simulink model "GateTestHarness_C"  (R2016a)
settings: Solver=FixedStepDiscrete  StartTime=0.0  StopTime=120  FixedStep=0.001  RelTol=1e-3
undefined symbols (not defined in the file or in its folder): sigbuilder_block
libraries: simulink x8
settings Model: Creator=omaro  LastModifiedBy=oelkawok
settings OptimizationCC: DefaultParameterBehavior=Inlined  OptimizeModelRefInitCode=on  LifeSpan=1
settings HardwareCC: ProdLongLongMode=on
settings RTWCC: SystemTargetFile=ert.tlc  TemplateMakefile=ert_default_tmf  GenerateReport=on  IncludeHyperlinkInReport=on  LaunchReport=on  GenerateTraceInfo=on  GenerateTraceReport=on  GenerateTraceReportSl=on  GenerateTraceReportSf=on  GenerateTraceReportEml=on
settings CodeAppCC: ForceParamTrailComments=on  IgnoreCustomStorageClasses=off  OperatorAnnotations=on  SimulinkDataObjDesc=on  SFDataObjDesc=on  MATLABFcnDesc=on  InsertBlockDesc=on  MATLABSourceComments=on
settings ERTTargetCC: GenerateSampleERTMain=on  InlinedParameterPlacement=NonHierarchical  ERTCustomFileTemplate=example_file_process.tlc

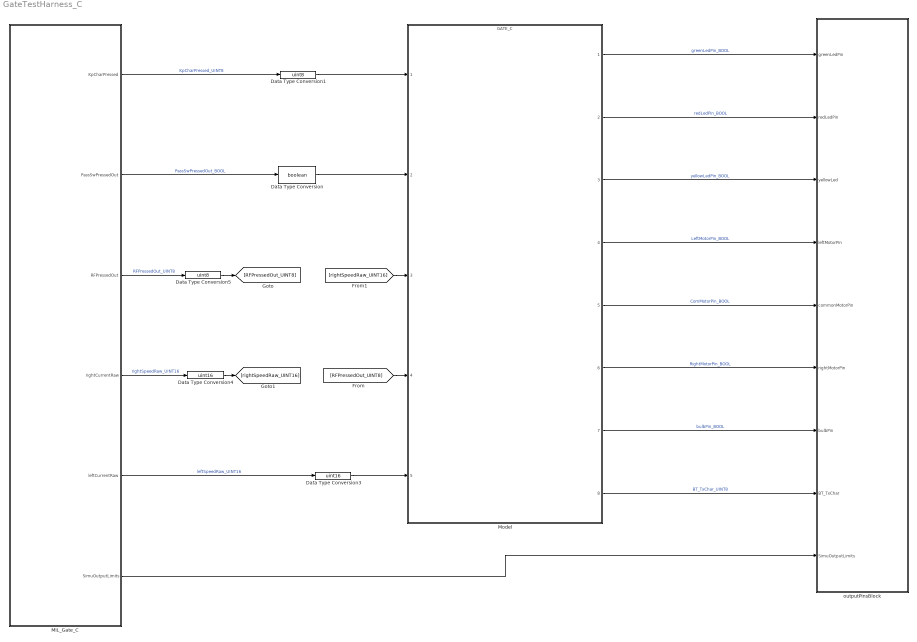
== system GateTestHarness_C ==
  Data Type Conversion : DataTypeConversion  OutDataTypeStr=boolean
  Data Type Conversion1 : DataTypeConversion  OutDataTypeStr=uint8
  Data Type Conversion3 : DataTypeConversion  OutDataTypeStr=uint16
  Data Type Conversion4 : DataTypeConversion  OutDataTypeStr=uint16
  Data Type Conversion5 : DataTypeConversion  OutDataTypeStr=uint8
  MIL_Gate_C : Subsystem  VariantControl=MIL_VariantC
  Model : ModelReference  ModelNameDialog=GATE_C.slx  SimulationMode=Normal  ModelReferenceVersion=1.328
  outputPinsBlock : Subsystem  Variant=on  VariantControl=Variant1  OverrideUsingVariant=VVOutputs
  wires:
  MIL_Gate_C/6(SimuOutputLimits) -> outputPinsBlock/9(SimuOutputLimits)
  Model/1 -> outputPinsBlock/1(greenLedPin)  "greenLedPin_BOOL"
  Model/2 -> outputPinsBlock/2(redLedPin)  "redLedPin_BOOL"
  Model/3 -> outputPinsBlock/3(yellowLed)  "yellowLedPin_BOOL"
  Model/4 -> outputPinsBlock/4(leftMotorPin)  "LeftMotorPin_BOOL"
  Model/5 -> outputPinsBlock/5(commonMotorPin)  "ComMotorPin_BOOL"
  Model/6 -> outputPinsBlock/6(rightMotorPin)  "RightMotorPin_BOOL"
  Model/7 -> outputPinsBlock/7(bulbPin)  "bulbPin_BOOL"
  Model/8 -> outputPinsBlock/8(BT_TxChar)  "BT_TxChar_UINT8"
  MIL_Gate_C/2(PassSwPressedOut) -> Data Type Conversion/1  "PassSwPressedOut_BOOL"
  MIL_Gate_C/4(rightCurrentRaw) -> Data Type Conversion4/1  "rightSpeedRaw_UINT16"
  MIL_Gate_C/3(RFPressedOut) -> Data Type Conversion5/1  "RFPressedOut_UINT8"
  MIL_Gate_C/5(leftCurrentRaw) -> Data Type Conversion3/1  "leftSpeedRaw_UINT16"
  MIL_Gate_C/1(KpCharPressed) -> Data Type Conversion1/1  "KpCharPressed_UINT8"
  Data Type Conversion1/1 -> Model/1
  Data Type Conversion3/1 -> Model/5
  Data Type Conversion/1 -> Model/2
  Data Type Conversion5/1 -> [RFPressedOut_UINT8]
  [RFPressedOut_UINT8] -> Model/4
  Data Type Conversion4/1 -> [rightSpeedRaw_UINT16]
  [rightSpeedRaw_UINT16] -> Model/3

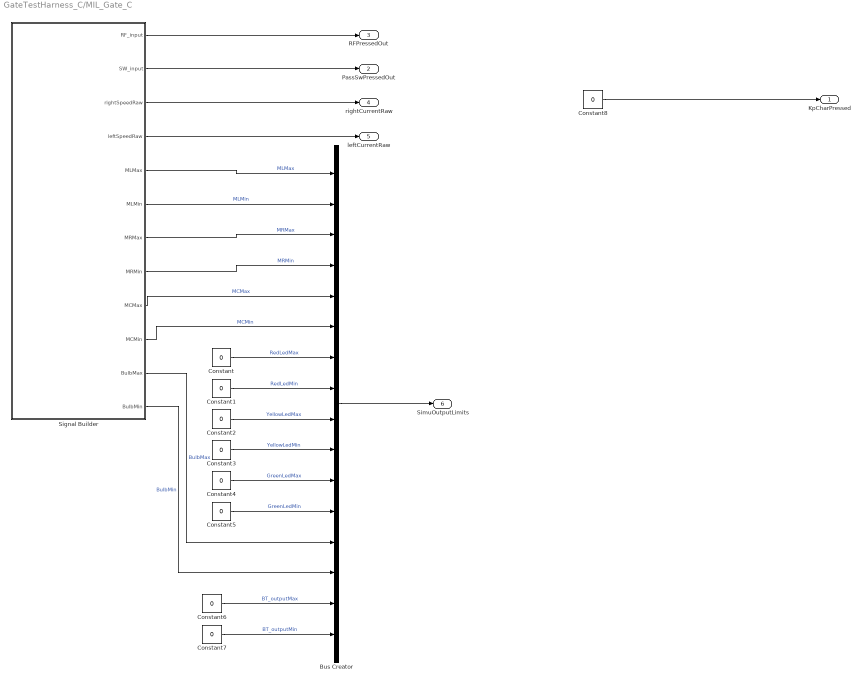
== system GateTestHarness_C/MIL_Gate_C ==
  Bus Creator : BusCreator  Inputs=16
  Constant{,1..8} (9 alike) : Constant  Value=0
  Signal Builder : Subsystem  Tag=STV Subsys  LoadFcn=sigbuilder_block('load',[588 31.2 565.2 553.2 ]);  StartFcn=sigbuilder_block('start');  StopFcn=sigbuilder_block('stop');  ClipboardFcn=sigbuilder_block('clipboard');  mask(Sigbuilder block){}
      mask help: Simulink:masks:SigbuilderBlock_MD
      mask init:
      | if ~strcmp(get_param(bdroot(gcbh),'SimulationStatus'),'stopped') tuvar = sigbuilder_block('maskInit'); end
      settings: CopyFcn=sigbuilder_block('copy');  DeleteFcn=sigbuilder_block('delete');  ModelCloseFcn=sigbuilder_block('modelClose');  PreSaveFcn=sigbuilder_block('preSave');  PauseFcn=sigbuilder_block('pause');  ContinueFcn=sigbuilder_block('continue');  NameChangeFcn=sigbuilder_block('namechange');  OpenFcn=sigbuilder_block('open',[6 6 1012.5 507 ]);  CloseFcn=sigbuilder_block('close');
      mask Display: plot(0, 0, 100, 100,[2, 2, 32, 32, 2], [68, 8, 8, 68, 68],[32, 2], [38, 38], [32, 19, 2],[53, 60, 44], [32, 17, 17, 2],[16, 16, 31, 31]);txt = getActiveGroup(gcbh);text(2, 100, txt,'verticalAlignment', 'top');
  KpCharPressed : Outport
  PassSwPressedOut : Outport  Port=2
  RFPressedOut : Outport  Port=3
  rightCurrentRaw : Outport  Port=4
  leftCurrentRaw : Outport  Port=5
  SimuOutputLimits : Outport  Port=6
  wires:
  Constant8/1 -> KpCharPressed/1
  Signal Builder/1(RF_input) -> RFPressedOut/1
  Signal Builder/2(SW_input) -> PassSwPressedOut/1
  Bus Creator/1 -> SimuOutputLimits/1
  Constant4/1 -> Bus Creator/11  "GreenLedMax"
  Constant3/1 -> Bus Creator/10  "YellowLedMin"
  Constant5/1 -> Bus Creator/12  "GreenLedMin"
  Constant2/1 -> Bus Creator/9  "YellowLedMax"
  Signal Builder/11(BulbMax) -> Bus Creator/13  "BulbMax"
  Constant1/1 -> Bus Creator/8  "RedLedMin"
  Signal Builder/12(BulbMin) -> Bus Creator/14  "BulbMin"
  Constant6/1 -> Bus Creator/15  "BT_outputMax"
  Constant/1 -> Bus Creator/7  "RedLedMax"
  Signal Builder/10(MCMin) -> Bus Creator/6  "MCMin"
  Signal Builder/9(MCMax) -> Bus Creator/5  "MCMax"
  Signal Builder/8(MRMin) -> Bus Creator/4  "MRMin"
  Signal Builder/7(MRMax) -> Bus Creator/3  "MRMax"
  Signal Builder/6(MLMin) -> Bus Creator/2  "MLMin"
  Signal Builder/5(MLMax) -> Bus Creator/1  "MLMax"
  Constant7/1 -> Bus Creator/16  "BT_outputMin"
  Signal Builder/3(rightSpeedRaw) -> rightCurrentRaw/1
  Signal Builder/4(leftSpeedRaw) -> leftCurrentRaw/1

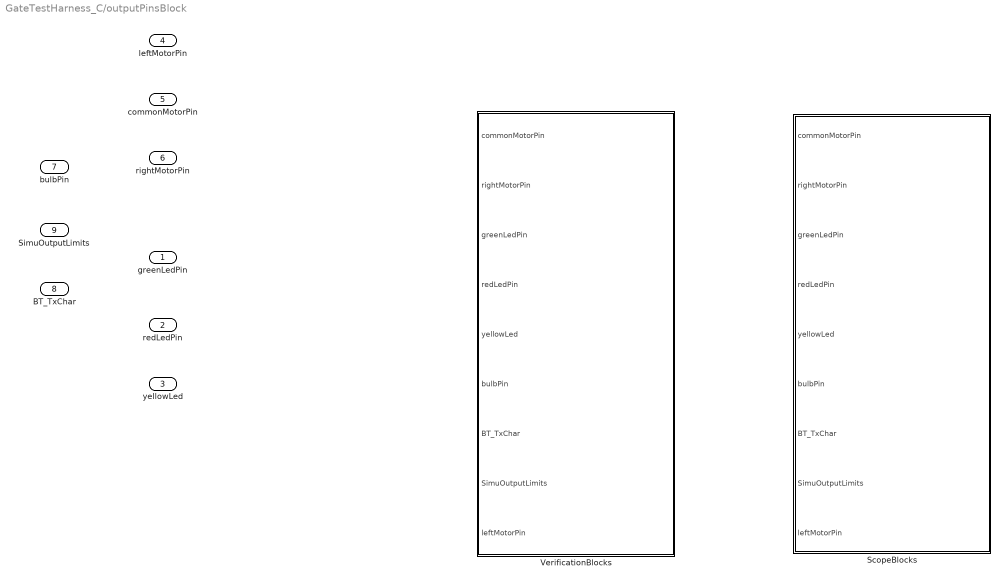
== system GateTestHarness_C/outputPinsBlock ==
  greenLedPin : Inport
  redLedPin : Inport  Port=2
  yellowLed : Inport  Port=3
  leftMotorPin : Inport  Port=4
  commonMotorPin : Inport  Port=5
  rightMotorPin : Inport  Port=6
  bulbPin : Inport  Port=7
  BT_TxChar : Inport  Port=8
  SimuOutputLimits : Inport  Port=9
  ScopeBlocks : Subsystem  VariantControl=VisualOutputs
  "VerificationBlocks " : Subsystem  VariantControl=VVOutputs

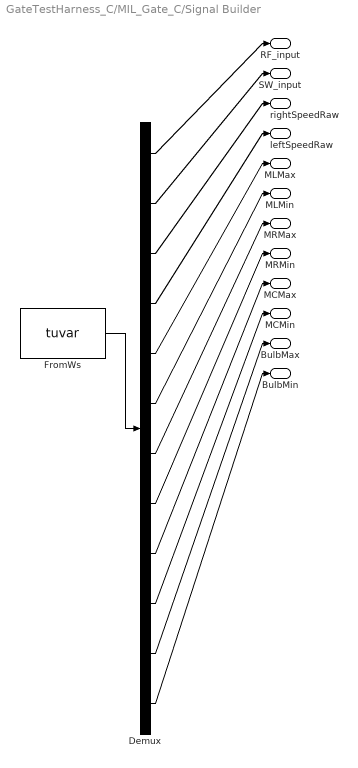
== system GateTestHarness_C/MIL_Gate_C/Signal Builder ==
  Demux : Demux  Tag=STV Demux  Outputs=12
  FromWs : FromWorkspace  Tag=STV FromWs  VariableName=tuvar  SampleTime=0
      SigBuilderData=|
      | common.afterFinalStr = 'Extrapolate'
      | common.sampleTime = 0
      | dataSet(1).timeRange = [0 120]
      | dataSet(1).name = 'RFinputOnly_C'
      | dataSet(2).timeRange = [0 120]
      | dataSet(2).name = 'RF_SW_input_C'
      | dataSet(3).timeRange = [0 120]
      | dataSet(3).name = 'SW_PauseBeforeSideDelay_C'
      | dataSet(4).timeRange = [0 120]
      | dataSet(4).name = 'SW_input2Cycles_C'
      | dataSet(5).timeRange = [0 120]
      | dataSet(5).name = 'RF_SW_inputOpeningTimeout_C'
      | sbobj.Groups(1).Name = 'RFinputOnly_C'
      | sbobj.Groups(1).Signals(1).Name = 'RF_input'
      | sbobj.Groups(1).Signals(1).XData = [0 3.85 3.85 4.01 4.01 31.15 31.15 31.347 31.347 120]
      | sbobj.Groups(1).Signals(1).YData = [0 0 1 1 0 0 1 1 0 0]
      | sbobj.Groups(1).Signals(2).Name = 'SW_input'
      | sbobj.Groups(1).Signals(2).XData = [0 120]
      | sbobj.Groups(1).Signals(2).YData = [0 0]
      | sbobj.Groups(1).Signals(3).Name = 'rightSpeedRaw'
      | sbobj.Groups(1).Signals(3).XData = [0 0.001 0.002 0.003 0.004 0.005 0.006 0.007 0.008 0.009 0.01 0.011 ... (120001 elements, 1x120001)]
      | sbobj.Groups(1).Signals(3).YData = [1023 1023 1023 1023 1023 1023 1023 1023 1023 1023 1023 1023 ... (120001 elements, 1x120001)]
      | sbobj.Groups(1).Signals(4).Name = 'leftSpeedRaw'
      | sbobj.Groups(1).Signals(4).XData = [0 0.001 0.002 0.003 0.004 0.005 0.006 0.007 0.008 0.009 0.01 0.011 ... (120001 elements, 1x120001)]
      | sbobj.Groups(1).Signals(4).YData = [1023 1023 1023 1023 1023 1023 1023 1023 1023 1023 1023 1023 ... (120001 elements, 1x120001)]
      | sbobj.Groups(1).Signals(5).Name = 'MLMax'
      | sbobj.Groups(1).Signals(5).XData = [0 3.5 3.5 19.5 19.5 31 31 35 35 120]
      | sbobj.Groups(1).Signals(5).YData = [0.1 0.1 1.1 1.1 0.1 0.1 1.1 1.1 0.1 0.1]
      | sbobj.Groups(1).Signals(6).Name = 'MLMin'
      | sbobj.Groups(1).Signals(6).XData = [0 4.05 4.05 17.4 17.4 31.5 31.5 33.6 33.6 120]
      | sbobj.Groups(1).Signals(6).YData = [-0.1 -0.1 0.9 0.9 -0.1 -0.1 0.9 0.9 -0.1 -0.1]
      | sbobj.Groups(1).Signals(7).Name = 'MRMax'
      | sbobj.Groups(1).Signals(7).XData = [0 6.75 6.75 19.5 19.5 30.35 120]
      | sbobj.Groups(1).Signals(7).YData = [0.1 0.1 1.1 1.1 0.1 0.1 0.1]
      | sbobj.Groups(1).Signals(8).Name = 'MRMin'
      | sbobj.Groups(1).Signals(8).XData = [0 7.55 7.55 18.5 18.5 120]
      | sbobj.Groups(1).Signals(8).YData = [-0.1 -0.1 0.9 0.9 -0.1 -0.1]
      | sbobj.Groups(1).Signals(9).Name = 'MCMax'
      | sbobj.Groups(1).Signals(9).XData = [0 31.9 31.9 46.2 46.2 120]
      | sbobj.Groups(1).Signals(9).YData = [1.1 1.1 0.1 0.1 1.1 1.1]
      | sbobj.Groups(1).Signals(10).Name = 'MCMin'
      | sbobj.Groups(1).Signals(10).XData = [0 31 31 47.7 47.7 120]
      | sbobj.Groups(1).Signals(10).YData = [0.9 0.9 -0.1 -0.1 0.9 0.9]
      | sbobj.Groups(1).Signals(11).Name = 'BulbMax'
      | sbobj.Groups(1).Signals(11).XData = [0 3.76 3.76 48.2 48.2 120]
      | sbobj.Groups(1).Signals(11).YData = [0.1 0.1 1.1 1.1 0.1 0.1]
      | sbobj.Groups(1).Signals(12).Name = 'BulbMin'
      | sbobj.Groups(1).Signals(12).XData = [0 4.27 4.27 46.2 46.2 120]
      | sbobj.Groups(1).Signals(12).YData = [-0.1 -0.1 0.9 0.9 -0.1 -0.1]
      | sbobj.Groups(1).TimeRange = [0 120]
      | sbobj.Groups(2).Name = 'RF_SW_input_C'
      | sbobj.Groups(2).Signals(1).Name = 'RF_input'
      | sbobj.Groups(2).Signals(1).XData = [0 3.85 3.85 4.01 4.01 120]
      | sbobj.Groups(2).Signals(1).YData = [0 0 1 1 0 0]
      | sbobj.Groups(2).Signals(2).Name = 'SW_input'
      | sbobj.Groups(2).Signals(2).XData = [0 31.17 31.17 31.65 31.65 120]
      | sbobj.Groups(2).Signals(2).YData = [0 0 1 1 0 0]
      | sbobj.Groups(2).Signals(3).Name = 'rightSpeedRaw'
      | sbobj.Groups(2).Signals(3).XData = [0 0.001 0.002 0.003 0.004 0.005 0.006 0.007 0.008 0.009 0.01 0.011 ... (120001 elements, 1x120001)]
      | sbobj.Groups(2).Signals(3).YData = [1023 1023 1023 1023 1023 1023 1023 1023 1023 1023 1023 1023 ... (120001 elements, 1x120001)]
      | sbobj.Groups(2).Signals(4).Name = 'leftSpeedRaw'
      | sbobj.Groups(2).Signals(4).XData = [0 0.001 0.002 0.003 0.004 0.005 0.006 0.007 0.008 0.009 0.01 0.011 ... (120001 elements, 1x120001)]
      | sbobj.Groups(2).Signals(4).YData = [1023 1023 1023 1023 1023 1023 1023 1023 1023 1023 1023 1023 ... (120001 elements, 1x120001)]
      | sbobj.Groups(2).Signals(5).Name = 'MLMax'
      | sbobj.Groups(2).Signals(5).XData = [0 3.5 3.5 19.5 19.5 31 31 35 35 120]
      | sbobj.Groups(2).Signals(5).YData = [0.1 0.1 1.1 1.1 0.1 0.1 1.1 1.1 0.1 0.1]
      | sbobj.Groups(2).Signals(6).Name = 'MLMin'
      | sbobj.Groups(2).Signals(6).XData = [0 4.05 4.05 18.5 18.5 31.5 31.5 33.8 33.8 120]
      | sbobj.Groups(2).Signals(6).YData = [-0.1 -0.1 0.9 0.9 -0.1 -0.1 0.9 0.9 -0.1 -0.1]
      | sbobj.Groups(2).Signals(7).Name = 'MRMax'
      | sbobj.Groups(2).Signals(7).XData = [0 6.75 6.75 19.5 19.5 30.35 120]
      | sbobj.Groups(2).Signals(7).YData = [0.1 0.1 1.1 1.1 0.1 0.1 0.1]
      | sbobj.Groups(2).Signals(8).Name = 'MRMin'
      | sbobj.Groups(2).Signals(8).XData = [0 7.55 7.55 18.5 18.5 120]
      | sbobj.Groups(2).Signals(8).YData = [-0.1 -0.1 0.9 0.9 -0.1 -0.1]
      | sbobj.Groups(2).Signals(9).Name = 'MCMax'
      | sbobj.Groups(2).Signals(9).XData = [0 31.9 31.9 46.2 46.2 120]
      | sbobj.Groups(2).Signals(9).YData = [1.1 1.1 0.1 0.1 1.1 1.1]
      | sbobj.Groups(2).Signals(10).Name = 'MCMin'
      | sbobj.Groups(2).Signals(10).XData = [0 31 31 47.7 47.7 120]
      | sbobj.Groups(2).Signals(10).YData = [0.9 0.9 -0.1 -0.1 0.9 0.9]
      | sbobj.Groups(2).Signals(11).Name = 'BulbMax'
      | sbobj.Groups(2).Signals(11).XData = [0 3.76 3.76 48.6 48.6 120]
      | sbobj.Groups(2).Signals(11).YData = [0.1 0.1 1.1 1.1 0.1 0.1]
      | sbobj.Groups(2).Signals(12).Name = 'BulbMin'
      | sbobj.Groups(2).Signals(12).XData = [0 4.27 4.27 46.2 46.2 120]
      | sbobj.Groups(2).Signals(12).YData = [-0.1 -0.1 0.9 0.9 -0.1 -0.1]
      | sbobj.Groups(2).TimeRange = [0 120]
      | sbobj.Groups(3).Name = 'SW_PauseBeforeSideDelay_C'
      | sbobj.Groups(3).Signals(1).Name = 'RF_input'
      | sbobj.Groups(3).Signals(1).XData = [0 120]
      | sbobj.Groups(3).Signals(1).YData = [0 0]
      | sbobj.Groups(3).Signals(2).Name = 'SW_input'
      | sbobj.Groups(3).Signals(2).XData = [0 3.88 3.88 4.55 4.55 5.5 5.5 6 6 11.35 11.35 12.1 12.1 31.17 31.17 31.65 31.65 120]
      | sbobj.Groups(3).Signals(2).YData = [0 0 1 1 0 0 1 1 0 0 1 1 0 0 1 1 0 0]
      | sbobj.Groups(3).Signals(3).Name = 'rightSpeedRaw'
      | sbobj.Groups(3).Signals(3).XData = [0 0.001 0.002 0.003 0.004 0.005 0.006 0.007 0.008 0.009 0.01 0.011 ... (120001 elements, 1x120001)]
      | sbobj.Groups(3).Signals(3).YData = [1023 1023 1023 1023 1023 1023 1023 1023 1023 1023 1023 1023 ... (120001 elements, 1x120001)]
      | sbobj.Groups(3).Signals(4).Name = 'leftSpeedRaw'
      | sbobj.Groups(3).Signals(4).XData = [0 0.001 0.002 0.003 0.004 0.005 0.006 0.007 0.008 0.009 0.01 0.011 ... (120001 elements, 1x120001)]
      | sbobj.Groups(3).Signals(4).YData = [1023 1023 1023 1023 1023 1023 1023 1023 1023 1023 1023 1023 ... (120001 elements, 1x120001)]
      | sbobj.Groups(3).Signals(5).Name = 'MLMax'
      | sbobj.Groups(3).Signals(5).XData = [0 3.5 3.5 12.5 12.5 31 31 35 35 120]
      | sbobj.Groups(3).Signals(5).YData = [0.1 0.1 1.1 1.1 0.1 0.1 1.1 1.1 0.1 0.1]
      | sbobj.Groups(3).Signals(6).Name = 'MLMin'
      | sbobj.Groups(3).Signals(6).XData = [0 4.05 4.05 10.6 10.6 31.5 31.5 33.8 33.8 120]
      | sbobj.Groups(3).Signals(6).YData = [-0.1 -0.1 0.9 0.9 -0.1 -0.1 0.9 0.9 -0.1 -0.1]
      | sbobj.Groups(3).Signals(7).Name = 'MRMax'
      | sbobj.Groups(3).Signals(7).XData = [0 6.75 6.75 12.9 12.9 30.35 120]
      | sbobj.Groups(3).Signals(7).YData = [0.1 0.1 1.1 1.1 0.1 0.1 0.1]
      | sbobj.Groups(3).Signals(8).Name = 'MRMin'
      | sbobj.Groups(3).Signals(8).XData = [0 7.55 7.55 10.4 10.4 120]
      | sbobj.Groups(3).Signals(8).YData = [-0.1 -0.1 0.9 0.9 -0.1 -0.1]
      | sbobj.Groups(3).Signals(9).Name = 'MCMax'
      | sbobj.Groups(3).Signals(9).XData = [0 31.9 31.9 46.2 46.2 120]
      | sbobj.Groups(3).Signals(9).YData = [1.1 1.1 0.1 0.1 1.1 1.1]
      | sbobj.Groups(3).Signals(10).Name = 'MCMin'
      | sbobj.Groups(3).Signals(10).XData = [0 31 31 47.7 47.7 120]
      | sbobj.Groups(3).Signals(10).YData = [0.9 0.9 -0.1 -0.1 0.9 0.9]
      | sbobj.Groups(3).Signals(11).Name = 'BulbMax'
      | sbobj.Groups(3).Signals(11).XData = [0 3.76 3.76 48.6 48.6 120]
      | sbobj.Groups(3).Signals(11).YData = [0.1 0.1 1.1 1.1 0.1 0.1]
      | sbobj.Groups(3).Signals(12).Name = 'BulbMin'
      | sbobj.Groups(3).Signals(12).XData = [0 4.27 4.27 46.2 46.2 120]
      | sbobj.Groups(3).Signals(12).YData = [-0.1 -0.1 0.9 0.9 -0.1 -0.1]
      | sbobj.Groups(3).TimeRange = [0 120]
      | sbobj.Groups(4).Name = 'SW_input2Cycles_C'
      | sbobj.Groups(4).Signals(1).Name = 'RF_input'
      | sbobj.Groups(4).Signals(1).XData = [0 23 23 23.2 23.2 120]
      | sbobj.Groups(4).Signals(1).YData = [0 0 1 1 0 0]
      | sbobj.Groups(4).Signals(2).Name = 'SW_input'
      | sbobj.Groups(4).Signals(2).XData = [0 3.85 3.85 4.1 4.1 43 43 43.88 43.88 79 79 80.14 80.14 120]
      | sbobj.Groups(4).Signals(2).YData = [0 0 1 1 0 0 1 1 0 0 1 1 0 0]
      | sbobj.Groups(4).Signals(3).Name = 'rightSpeedRaw'
      | sbobj.Groups(4).Signals(3).XData = [0 0.001 0.002 0.003 0.004 0.005 0.006 0.007 0.008 0.009 0.01 0.011 ... (120001 elements, 1x120001)]
      | sbobj.Groups(4).Signals(3).YData = [1023 1023 1023 1023 1023 1023 1023 1023 1023 1023 1023 1023 ... (120001 elements, 1x120001)]
      | sbobj.Groups(4).Signals(4).Name = 'leftSpeedRaw'
      | sbobj.Groups(4).Signals(4).XData = [0 0.001 0.002 0.003 0.004 0.005 0.006 0.007 0.008 0.009 0.01 0.011 ... (120001 elements, 1x120001)]
      | sbobj.Groups(4).Signals(4).YData = [1023 1023 1023 1023 1023 1023 1023 1023 1023 1023 1023 1023 ... (120001 elements, 1x120001)]
      | sbobj.Groups(4).Signals(5).Name = 'MLMax'
      | sbobj.Groups(4).Signals(5).XData = [0 3.5 3.5 19.5 19.5 22.5 22.5 26.5 26.5 42.5 42.5 58.5 58.5 78.5 78.5 82.5 82.5 120]
      | sbobj.Groups(4).Signals(5).YData = [0.1 0.1 1.1 1.1 0.1 0.1 1.1 1.1 0.1 0.1 1.1 1.1 0.1 0.1 1.1 1.1 0.1 0.1]
      | sbobj.Groups(4).Signals(6).Name = 'MLMin'
      | sbobj.Groups(4).Signals(6).XData = [0 4.05 4.05 18.5 18.5 23.5 23.5 25.5 25.5 43.5 43.5 57.5 57.5 79.5 79.5 81.5 81.5 120]
      | sbobj.Groups(4).Signals(6).YData = [-0.1 -0.1 0.9 0.9 -0.1 -0.1 0.9 0.9 -0.1 -0.1 0.9 0.9 -0.1 -0.1 0.9 0.9 -0.1 -0.1]
      | sbobj.Groups(4).Signals(7).Name = 'MRMax'
      | sbobj.Groups(4).Signals(7).XData = [0 6.75 6.75 19.5 19.5 45.5 45.5 58.5 58.5 120]
      | sbobj.Groups(4).Signals(7).YData = [0.1 0.1 1.1 1.1 0.1 0.1 1.1 1.1 0.1 0.1]
      | sbobj.Groups(4).Signals(8).Name = 'MRMin'
      | sbobj.Groups(4).Signals(8).XData = [0 7.55 7.55 18.5 18.5 46.5 46.5 57.5 57.5 120]
      | sbobj.Groups(4).Signals(8).YData = [-0.1 -0.1 0.9 0.9 -0.1 -0.1 0.9 0.9 -0.1 -0.1]
      | sbobj.Groups(4).Signals(9).Name = 'MCMax'
      | sbobj.Groups(4).Signals(9).XData = [0 23.5 23.5 37.5 37.5 79.5 79.5 93.5 93.5 120]
      | sbobj.Groups(4).Signals(9).YData = [1.1 1.1 0.1 0.1 1.1 1.1 0.1 0.1 1.1 1.1]
      | sbobj.Groups(4).Signals(10).Name = 'MCMin'
      | sbobj.Groups(4).Signals(10).XData = [0 22.5 22.5 38.5 38.5 78.5 78.5 94.5 94.5 120]
      | sbobj.Groups(4).Signals(10).YData = [0.9 0.9 -0.1 -0.1 0.9 0.9 -0.1 -0.1 0.9 0.9]
      | sbobj.Groups(4).Signals(11).Name = 'BulbMax'
      | sbobj.Groups(4).Signals(11).XData = [0 3.76 3.76 38.9 38.9 42.5 42.5 94.5 94.5 120]
      | sbobj.Groups(4).Signals(11).YData = [0.1 0.1 1.1 1.1 0.1 0.1 1.1 1.1 0.1 0.1]
      | sbobj.Groups(4).Signals(12).Name = 'BulbMin'
      | sbobj.Groups(4).Signals(12).XData = [0 4.27 4.27 37.9 37.9 43.5 43.5 93.5 93.5 120]
      | sbobj.Groups(4).Signals(12).YData = [-0.1 -0.1 0.9 0.9 -0.1 -0.1 0.9 0.9 -0.1 -0.1]
      | sbobj.Groups(4).TimeRange = [0 120]
      | sbobj.Groups(5).Name = 'RF_SW_inputOpeningTimeout_C'
      | sbobj.Groups(5).Signals(1).Name = 'RF_input'
      | sbobj.Groups(5).Signals(1).XData = [0 3.85 3.85 4.01 4.01 120]
      | sbobj.Groups(5).Signals(1).YData = [0 0 1 1 0 0]
      | sbobj.Groups(5).Signals(2).Name = 'SW_input'
      | sbobj.Groups(5).Signals(2).XData = [0 45.05 45.05 46.25 46.25 120]
      | sbobj.Groups(5).Signals(2).YData = [0 0 1 1 0 0]
      | sbobj.Groups(5).Signals(3).Name = 'rightSpeedRaw'
      | sbobj.Groups(5).Signals(3).XData = [0 0.001 0.002 0.003 0.004 0.005 0.006 0.007 0.008 0.009 0.01 0.011 ... (120001 elements, 1x120001)]
      | sbobj.Groups(5).Signals(3).YData = [1023 1023 1023 1023 1023 1023 1023 1023 1023 1023 1023 1023 ... (120001 elements, 1x120001)]
      | sbobj.Groups(5).Signals(4).Name = 'leftSpeedRaw'
      | sbobj.Groups(5).Signals(4).XData = [0 0.001 0.002 0.003 0.004 0.005 0.006 0.007 0.008 0.009 0.01 0.011 ... (120001 elements, 1x120001)]
      | sbobj.Groups(5).Signals(4).YData = [1023 1023 1023 1023 1023 1023 1023 1023 1023 1023 1023 1023 ... (120001 elements, 1x120001)]
      | sbobj.Groups(5).Signals(5).Name = 'MLMax'
      | sbobj.Groups(5).Signals(5).XData = [0 3.5 3.5 35.5 35.5 44 44 48.6 48.6 120]
      | sbobj.Groups(5).Signals(5).YData = [0.1 0.1 1.1 1.1 0.1 0.1 1.1 1.1 0.1 0.1]
      | sbobj.Groups(5).Signals(6).Name = 'MLMin'
      | sbobj.Groups(5).Signals(6).XData = [0 4.05 4.05 33.5 33.5 45.6 45.6 47.2 47.2 120]
      | sbobj.Groups(5).Signals(6).YData = [-0.1 -0.1 0.9 0.9 -0.1 -0.1 0.9 0.9 -0.1 -0.1]
      | sbobj.Groups(5).Signals(7).Name = 'MRMax'
      | sbobj.Groups(5).Signals(7).XData = [0 6.75 6.75 35.6 35.6 120]
      | sbobj.Groups(5).Signals(7).YData = [0.1 0.1 1.1 1.1 0.1 0.1]
      | sbobj.Groups(5).Signals(8).Name = 'MRMin'
      | sbobj.Groups(5).Signals(8).XData = [0 7.55 7.55 33.7 33.7 120]
      | sbobj.Groups(5).Signals(8).YData = [-0.1 -0.1 0.9 0.9 -0.1 -0.1]
      | sbobj.Groups(5).Signals(9).Name = 'MCMax'
      | sbobj.Groups(5).Signals(9).XData = [0 45.9 45.9 59.3 59.3 120]
      | sbobj.Groups(5).Signals(9).YData = [1.1 1.1 0.1 0.1 1.1 1.1]
      | sbobj.Groups(5).Signals(10).Name = 'MCMin'
      | sbobj.Groups(5).Signals(10).XData = [0 44.6 44.6 60.6 60.6 120]
      | sbobj.Groups(5).Signals(10).YData = [0.9 0.9 -0.1 -0.1 0.9 0.9]
      | sbobj.Groups(5).Signals(11).Name = 'BulbMax'
      | sbobj.Groups(5).Signals(11).XData = [0 3.76 3.76 60.8 60.8 120]
      | sbobj.Groups(5).Signals(11).YData = [0.1 0.1 1.1 1.1 0.1 0.1]
      | sbobj.Groups(5).Signals(12).Name = 'BulbMin'
      | sbobj.Groups(5).Signals(12).XData = [0 4.27 4.27 59.4 59.4 120]
      | sbobj.Groups(5).Signals(12).YData = [-0.1 -0.1 0.9 0.9 -0.1 -0.1]
      | sbobj.Groups(5).TimeRange = [0 120]
  RF_input : Outport  Tag=STV Outport
  SW_input : Outport  Tag=STV Outport  Port=2
  rightSpeedRaw : Outport  Tag=STV Outport  Port=3
  leftSpeedRaw : Outport  Tag=STV Outport  Port=4
  MLMax : Outport  Tag=STV Outport  Port=5
  MLMin : Outport  Tag=STV Outport  Port=6
  MRMax : Outport  Tag=STV Outport  Port=7
  MRMin : Outport  Tag=STV Outport  Port=8
  MCMax : Outport  Tag=STV Outport  Port=9
  MCMin : Outport  Tag=STV Outport  Port=10
  BulbMax : Outport  Tag=STV Outport  Port=11
  BulbMin : Outport  Tag=STV Outport  Port=12
  wires:
  FromWs/1 -> Demux/1
  Demux/1 -> RF_input/1
  Demux/2 -> SW_input/1
  Demux/3 -> rightSpeedRaw/1
  Demux/4 -> leftSpeedRaw/1
  Demux/5 -> MLMax/1
  Demux/6 -> MLMin/1
  Demux/7 -> MRMax/1
  Demux/8 -> MRMin/1
  Demux/9 -> MCMax/1
  Demux/10 -> MCMin/1
  Demux/11 -> BulbMax/1
  Demux/12 -> BulbMin/1

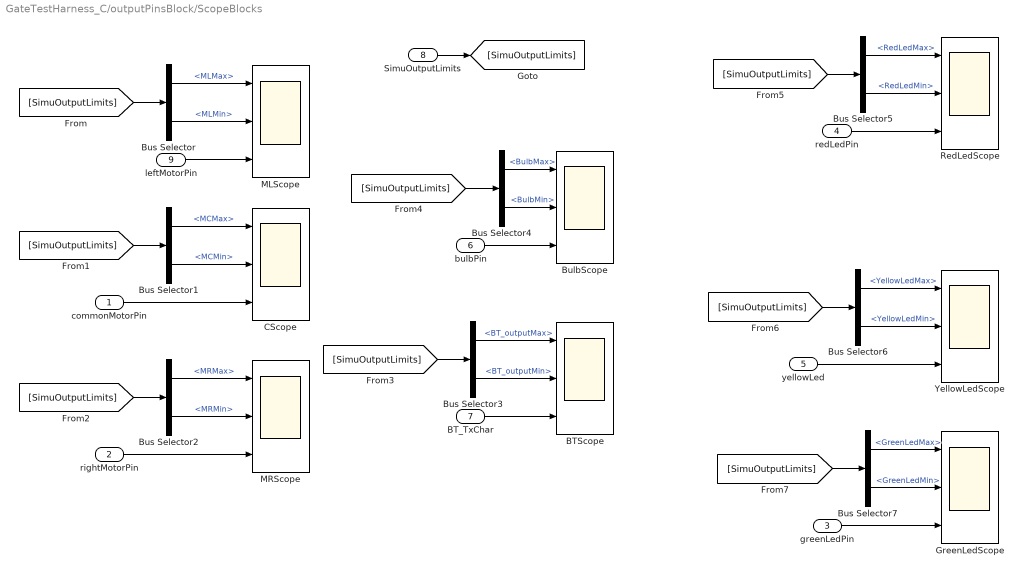
== system GateTestHarness_C/outputPinsBlock/ScopeBlocks ==
  commonMotorPin : Inport
  rightMotorPin : Inport  Port=2
  greenLedPin : Inport  Port=3
  redLedPin : Inport  Port=4
  yellowLed : Inport  Port=5
  bulbPin : Inport  Port=6
  BT_TxChar : Inport  Port=7
  SimuOutputLimits : Inport  Port=8
  leftMotorPin : Inport  Port=9
  BTScope : Scope  NumInputPorts=3
  BulbScope : Scope  NumInputPorts=3
  Bus Selector : BusSelector  OutputSignals=MLMax,MLMin
  Bus Selector1 : BusSelector  OutputSignals=MCMax,MCMin
  Bus Selector2 : BusSelector  OutputSignals=MRMax,MRMin
  Bus Selector3 : BusSelector  OutputSignals=BT_outputMax,BT_outputMin
  Bus Selector4 : BusSelector  OutputSignals=BulbMax,BulbMin
  Bus Selector5 : BusSelector  OutputSignals=RedLedMax,RedLedMin
  Bus Selector6 : BusSelector  OutputSignals=YellowLedMax,YellowLedMin
  Bus Selector7 : BusSelector  OutputSignals=GreenLedMax,GreenLedMin
  CScope : Scope  NumInputPorts=3
  GreenLedScope : Scope  NumInputPorts=3
  MLScope : Scope  NumInputPorts=3
  MRScope : Scope  NumInputPorts=3
  RedLedScope : Scope  NumInputPorts=3
  YellowLedScope : Scope  NumInputPorts=3
  wires:
  rightMotorPin/1 -> MRScope/3
  commonMotorPin/1 -> CScope/3
  bulbPin/1 -> BulbScope/3
  greenLedPin/1 -> GreenLedScope/3
  yellowLed/1 -> YellowLedScope/3
  redLedPin/1 -> RedLedScope/3
  BT_TxChar/1 -> BTScope/3
  SimuOutputLimits/1 -> [SimuOutputLimits]
  [SimuOutputLimits] -> Bus Selector/1
  leftMotorPin/1 -> MLScope/3
  Bus Selector/1 -> MLScope/1  "<MLMax>"
  Bus Selector/2 -> MLScope/2  "<MLMin>"
  [SimuOutputLimits] -> Bus Selector1/1
  Bus Selector1/1 -> CScope/1  "<MCMax>"
  Bus Selector1/2 -> CScope/2  "<MCMin>"
  [SimuOutputLimits] -> Bus Selector2/1
  Bus Selector2/1 -> MRScope/1  "<MRMax>"
  Bus Selector2/2 -> MRScope/2  "<MRMin>"
  [SimuOutputLimits] -> Bus Selector3/1
  Bus Selector3/1 -> BTScope/1  "<BT_outputMax>"
  Bus Selector3/2 -> BTScope/2  "<BT_outputMin>"
  [SimuOutputLimits] -> Bus Selector4/1
  Bus Selector4/1 -> BulbScope/1  "<BulbMax>"
  Bus Selector4/2 -> BulbScope/2  "<BulbMin>"
  [SimuOutputLimits] -> Bus Selector5/1
  Bus Selector5/1 -> RedLedScope/1  "<RedLedMax>"
  Bus Selector5/2 -> RedLedScope/2  "<RedLedMin>"
  [SimuOutputLimits] -> Bus Selector6/1
  Bus Selector6/1 -> YellowLedScope/1  "<YellowLedMax>"
  Bus Selector6/2 -> YellowLedScope/2  "<YellowLedMin>"
  [SimuOutputLimits] -> Bus Selector7/1
  Bus Selector7/1 -> GreenLedScope/1  "<GreenLedMax>"
  Bus Selector7/2 -> GreenLedScope/2  "<GreenLedMin>"

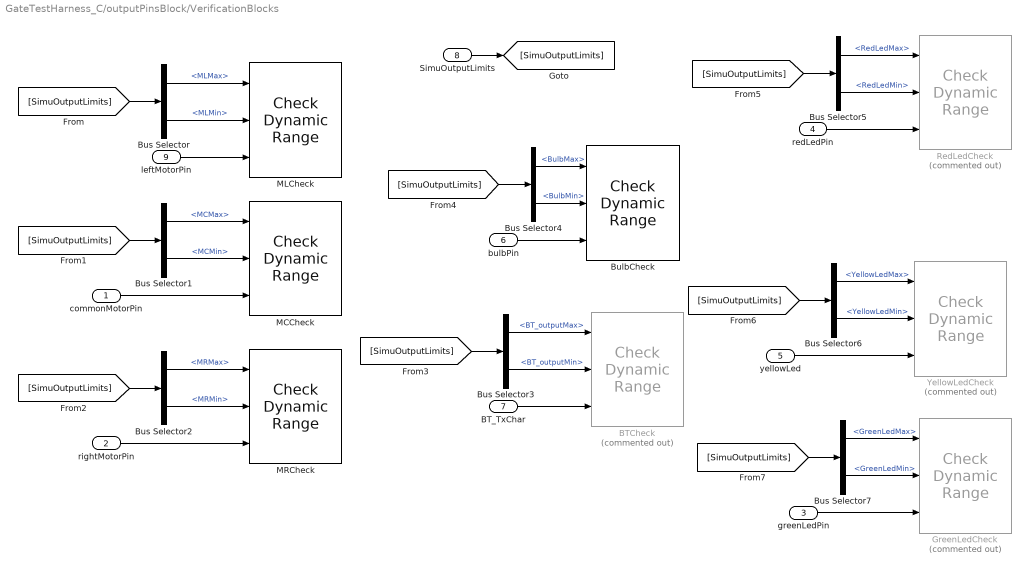
== system GateTestHarness_C/outputPinsBlock/VerificationBlocks  ==
  commonMotorPin : Inport
  rightMotorPin : Inport  Port=2
  greenLedPin : Inport  Port=3
  redLedPin : Inport  Port=4
  yellowLed : Inport  Port=5
  bulbPin : Inport  Port=6
  BT_TxChar : Inport  Port=7
  SimuOutputLimits : Inport  Port=8
  leftMotorPin : Inport  Port=9
  BTCheck : simulink/Model Verification/Check  Dynamic Range  Description=min < sig < max  Commented=on  enabled=on  stopWhenAssertionFail=on  export=off  icon=graphic
  BulbCheck : simulink/Model Verification/Check  Dynamic Range  Description=min < sig < max  enabled=on  stopWhenAssertionFail=on  export=off  icon=graphic
  Bus Selector : BusSelector  OutputSignals=MLMax,MLMin
  Bus Selector1 : BusSelector  OutputSignals=MCMax,MCMin
  Bus Selector2 : BusSelector  OutputSignals=MRMax,MRMin
  Bus Selector3 : BusSelector  OutputSignals=BT_outputMax,BT_outputMin
  Bus Selector4 : BusSelector  OutputSignals=BulbMax,BulbMin
  Bus Selector5 : BusSelector  OutputSignals=RedLedMax,RedLedMin
  Bus Selector6 : BusSelector  OutputSignals=YellowLedMax,YellowLedMin
  Bus Selector7 : BusSelector  OutputSignals=GreenLedMax,GreenLedMin
  GreenLedCheck : simulink/Model Verification/Check  Dynamic Range  Description=min < sig < max  Commented=on  enabled=on  stopWhenAssertionFail=on  export=off  icon=graphic
  MCCheck : simulink/Model Verification/Check  Dynamic Range  Description=min < sig < max  enabled=on  stopWhenAssertionFail=on  export=off  icon=graphic
  MLCheck : simulink/Model Verification/Check  Dynamic Range  Description=min < sig < max  enabled=on  stopWhenAssertionFail=on  export=off  icon=graphic
  MRCheck : simulink/Model Verification/Check  Dynamic Range  Description=min < sig < max  enabled=on  stopWhenAssertionFail=on  export=off  icon=graphic
  RedLedCheck : simulink/Model Verification/Check  Dynamic Range  Description=min < sig < max  Commented=on  enabled=on  stopWhenAssertionFail=on  export=off  icon=graphic
  YellowLedCheck : simulink/Model Verification/Check  Dynamic Range  Description=min < sig < max  Commented=on  enabled=on  stopWhenAssertionFail=on  export=off  icon=graphic
  wires:
  rightMotorPin/1 -> MRCheck/3
  commonMotorPin/1 -> MCCheck/3
  bulbPin/1 -> BulbCheck/3
  greenLedPin/1 -> GreenLedCheck/3
  yellowLed/1 -> YellowLedCheck/3
  redLedPin/1 -> RedLedCheck/3
  BT_TxChar/1 -> BTCheck/3
  SimuOutputLimits/1 -> [SimuOutputLimits]
  [SimuOutputLimits] -> Bus Selector/1
  leftMotorPin/1 -> MLCheck/3
  Bus Selector/1 -> MLCheck/1  "<MLMax>"
  Bus Selector/2 -> MLCheck/2  "<MLMin>"
  [SimuOutputLimits] -> Bus Selector1/1
  Bus Selector1/1 -> MCCheck/1  "<MCMax>"
  Bus Selector1/2 -> MCCheck/2  "<MCMin>"
  [SimuOutputLimits] -> Bus Selector2/1
  Bus Selector2/1 -> MRCheck/1  "<MRMax>"
  Bus Selector2/2 -> MRCheck/2  "<MRMin>"
  [SimuOutputLimits] -> Bus Selector3/1
  Bus Selector3/1 -> BTCheck/1  "<BT_outputMax>"
  Bus Selector3/2 -> BTCheck/2  "<BT_outputMin>"
  [SimuOutputLimits] -> Bus Selector4/1
  Bus Selector4/1 -> BulbCheck/1  "<BulbMax>"
  Bus Selector4/2 -> BulbCheck/2  "<BulbMin>"
  [SimuOutputLimits] -> Bus Selector5/1
  Bus Selector5/1 -> RedLedCheck/1  "<RedLedMax>"
  Bus Selector5/2 -> RedLedCheck/2  "<RedLedMin>"
  [SimuOutputLimits] -> Bus Selector6/1
  Bus Selector6/1 -> YellowLedCheck/1  "<YellowLedMax>"
  Bus Selector6/2 -> YellowLedCheck/2  "<YellowLedMin>"
  [SimuOutputLimits] -> Bus Selector7/1
  Bus Selector7/1 -> GreenLedCheck/1  "<GreenLedMax>"
  Bus Selector7/2 -> GreenLedCheck/2  "<GreenLedMin>"
